simulink model "designCheck"  (R2018b)
settings: Solver=VariableStepAuto  StartTime=0.0  StopTime=100  RelTol=1e-3
values from neighbouring files (symbols this model uses):
  plane = AirPlane("NT-33A_4.xlsx")    [entryPoint.m]    (also in main.m)
  servo = tf(10,[1 10])    [main.m]
libraries: simulink_extras x4, cstblocks x2
settings Model: Creator=OWNER  LastModifiedBy=OWNER

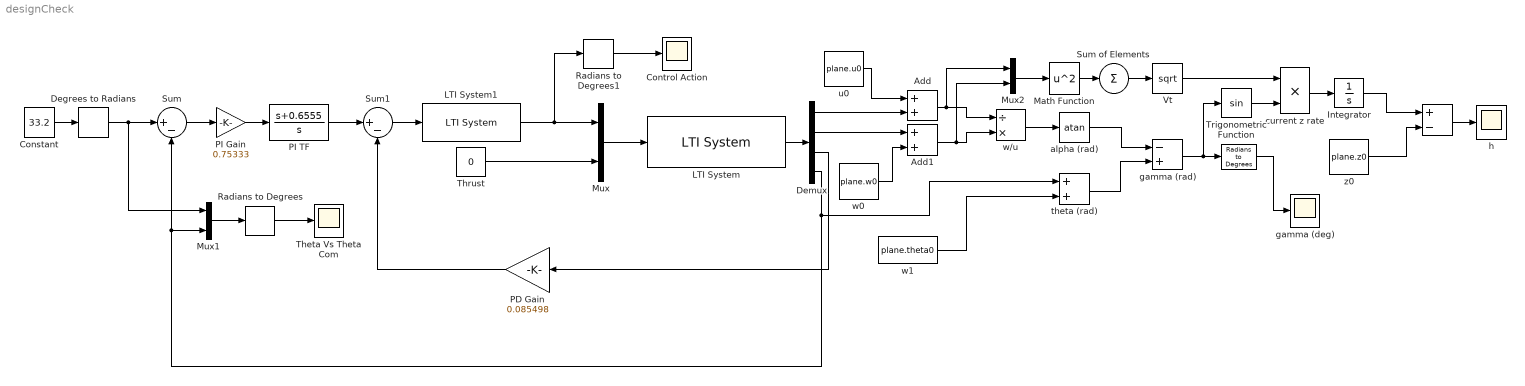
== system designCheck ==
  " " : simulink_extras/Transformations/Radians to Degrees
  "  " : Sum  Inputs=+-
  Add : Sum
  Add1 : Sum
  Constant : Constant  Value=33.2
  Control Action : Scope
  Degrees to Radians : simulink_extras/Transformations/Degrees to Radians
  Demux : Demux
  Integrator : Integrator
  LTI System : cstblocks/LTI System  sys=LongSS  IC=[]
  LTI System1 : cstblocks/LTI System  sys=-servo  IC=[]
  Math Function : Math  Operator=square  SaturateOnIntegerOverflow=on
  Mux : Mux  Inputs=2
  Mux1 : Mux  Inputs=2
  Mux2 : Mux  Inputs=2
  PD Gain : Gain  Gain=0.085498
  PI Gain : Gain  Gain=0.75333
  PI TF : TransferFcn  Numerator=[1 0.6555]  Denominator=[1 0]
  Radians to Degrees : simulink_extras/Transformations/Radians to Degrees
  Radians to Degrees1 : simulink_extras/Transformations/Radians to Degrees
  Sum : Sum  Inputs=|+-
  Sum of Elements : Sum  Inputs=+
  Sum1 : Sum  Inputs=|+-
  Theta Vs Theta Com : Scope
  Thrust : Constant  Value=0
  Trigonometric Function : Trigonometry
  Vt : Sqrt  SaturateOnIntegerOverflow=on
  alpha (rad) : Trigonometry  Operator=atan
  current z rate : Product
  gamma (deg) : Scope
  gamma (rad) : Sum  Inputs=-+
  h : Scope
  theta (rad) : Sum
  u0 : Constant  Value=plane.u0
  w/u : Product  Inputs=/*
  w0 : Constant  Value=plane.w0
  w1 : Constant  Value=plane.theta0
  z0 : Constant  Value=plane.z0
  wires:
  LTI System/1 -> Demux/1
  Mux/1 -> LTI System/1
  LTI System1/1 -> Radians to Degrees1/1, Mux/1
  Constant/1 -> Degrees to Radians/1
  Degrees to Radians/1 -> Mux1/1, Sum/1
  Demux/4 -> Mux1/2, Sum/2, theta (rad)/1
  Sum/1 -> PI Gain/1
  PI Gain/1 -> PI TF/1
  PI TF/1 -> Sum1/1
  Sum1/1 -> LTI System1/1
  Demux/3 -> PD Gain/1
  PD Gain/1 -> Sum1/2
  Thrust/1 -> Mux/2
  Radians to Degrees1/1 -> Control Action/1
  Radians to Degrees/1 -> Theta Vs Theta Com/1
  Mux1/1 -> Radians to Degrees/1
  Demux/1 -> Add/2
  u0/1 -> Add/1
  Demux/2 -> Add1/1
  w0/1 -> Add1/2
  Add1/1 -> Mux2/2, w/u/2
  Add/1 -> Mux2/1, w/u/1
  w/u/1 -> alpha (rad)/1
  w1/1 -> theta (rad)/2
  alpha (rad)/1 -> gamma (rad)/1
  theta (rad)/1 -> gamma (rad)/2
  gamma (rad)/1 -> Trigonometric Function/1, " "/1
  " "/1 -> gamma (deg)/1
  Mux2/1 -> Math Function/1
  Math Function/1 -> Sum of Elements/1
  Sum of Elements/1 -> Vt/1
  Vt/1 -> current z rate/1
  Trigonometric Function/1 -> current z rate/2
  current z rate/1 -> Integrator/1
  Integrator/1 -> "  "/1
  "  "/1 -> h/1
  z0/1 -> "  "/2
